simulink model "task_5_sim"  (R2022b)
settings: Solver=VariableStepAuto  StartTime=0.0  StopTime=20.0  RelTol=1e-3
model workspace (MAT data in the model file):
  C0 = [1  0  0  0  0  0; 0  1  0  0  0  0; 0  0  1  0  0  0; 0  0  0  1  0  0; 0  0  0  0  1  0; 0  0  0  0  0  1]
  D0 = [0  0; 0  0; 0  0; 0  0; 0  0; 0  0]
values from neighbouring files (symbols this model uses):
  KTld5_1 = real(getLQRController(ATld, BTld, Q, R))    [task5.m]
  L5_1 = K5_1'    [task5.m]
  r = -1/10*C*inv(A)*B*[-0.5+(a-b)/20; 0.1+(b-c)/(a+d+10)]    [task5.m]
undefined symbols (not defined in the file or in its folder): A, B, C
settings Model: Creator=小灰  LastModifiedBy=小灰

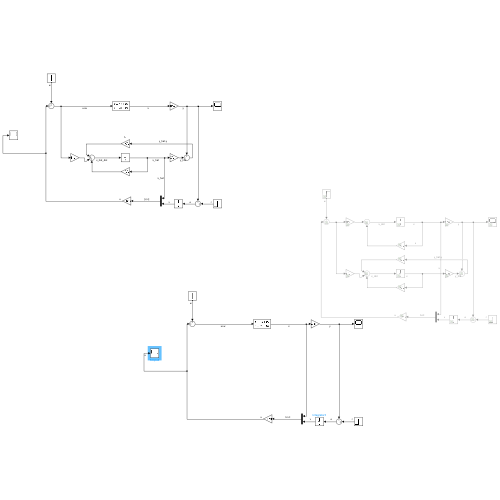
[thumbnail: Simulink's stored preview of the top-level diagram]
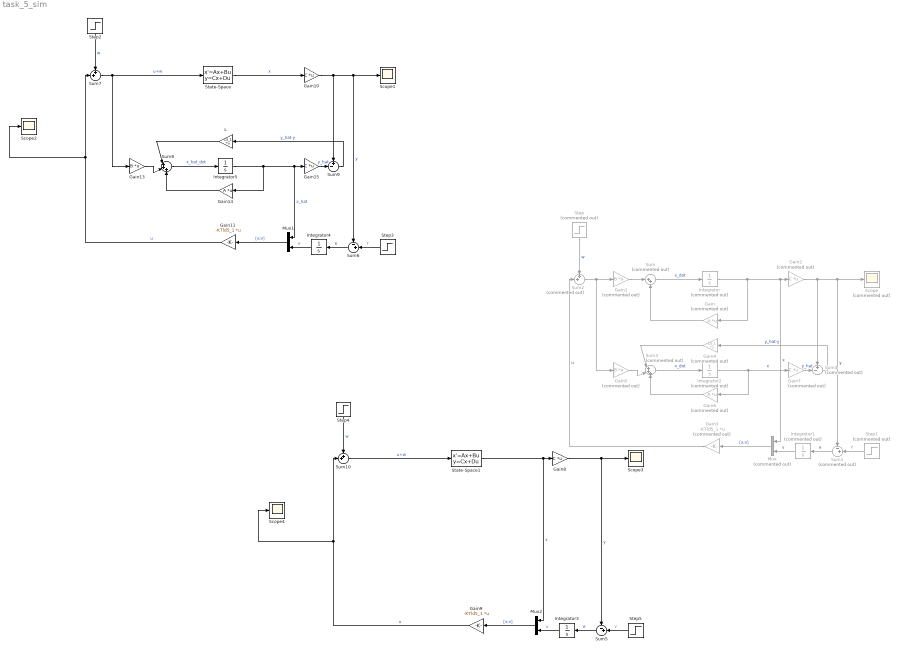
== system task_5_sim ==
  Gain : Gain  Commented=on  Gain=A  Multiplication=Matrix(K*u)
  Gain1 : Gain  Commented=on  Gain=B  Multiplication=Matrix(K*u)
  Gain10 : Gain  Gain=C  Multiplication=Matrix(K*u)
  Gain11 : Gain  Gain=-KTld5_1  Multiplication=Matrix(K*u)
  Gain13 : Gain  Gain=B  Multiplication=Matrix(K*u)
  Gain14 : Gain  Gain=A  Multiplication=Matrix(K*u)
  Gain15 : Gain  Gain=C  Multiplication=Matrix(K*u)
  Gain2 : Gain  Commented=on  Gain=C  Multiplication=Matrix(K*u)
  Gain3 : Gain  Commented=on  Gain=-KTld5_1  Multiplication=Matrix(K*u)
  Gain4 : Gain  Commented=on  Gain=L5_1  Multiplication=Matrix(K*u)
  Gain5 : Gain  Commented=on  Gain=B  Multiplication=Matrix(K*u)
  Gain6 : Gain  Commented=on  Gain=A  Multiplication=Matrix(K*u)
  Gain7 : Gain  Commented=on  Gain=C  Multiplication=Matrix(K*u)
  Gain8 : Gain  Gain=C  Multiplication=Matrix(K*u)
  Gain9 : Gain  Gain=-KTld5_1  Multiplication=Matrix(K*u)
  Integrator : Integrator  Commented=on
  Integrator1 : Integrator  Commented=on
  Integrator2 : Integrator  Commented=on
  Integrator3 : Integrator
  Integrator4 : Integrator
  Integrator5 : Integrator
  L : Gain  Gain=L5_1  Multiplication=Matrix(K*u)
  Mux : Mux  Commented=on  Inputs=2
  Mux1 : Mux  Inputs=2
  Mux2 : Mux  Inputs=2
  Scope : Scope  Commented=on
  Scope{1..4} (4 alike) : Scope
  State-Space : StateSpace  A=A  B=B  C=C0  D=D0  InitialCondition=0
  State-Space1 : StateSpace  A=A  B=B  C=C0  D=D0  InitialCondition=0
  Step : Step  Commented=on  Time=10  Before=[0;0]  After=[0;0]  SampleTime=0
  Step1 : Step  Commented=on  After=[0;1;0]  SampleTime=0
  Step2 : Step  Time=10  Before=[0;0]  After=0  SampleTime=0
  Step3 : Step  After=r  SampleTime=0
  Step4 : Step  Time=10  Before=[0;0]  After=0  SampleTime=0
  Step5 : Step  After=r  SampleTime=0
  Sum : Sum  Commented=on  Inputs=|++
  Sum1 : Sum  Commented=on  Inputs=-+|
  Sum10 : Sum  Inputs=++|
  Sum2 : Sum  Commented=on  Inputs=++|
  Sum3 : Sum  Commented=on  Inputs=|+++
  Sum4 : Sum  Commented=on  Inputs=+-|
  Sum5 : Sum  Inputs=-+|
  Sum6 : Sum  Inputs=-+|
  Sum7 : Sum  Inputs=++|
  Sum8 : Sum  Inputs=|+++
  Sum9 : Sum  Inputs=+-|
  wires:
  Sum/1 -> Integrator/1  "x_dot"
  Integrator/1 -> Gain/1, Mux/1, Gain2/1  "x"
  Gain2/1 -> Sum1/1, Scope/1, Sum4/1  "y"
  Mux/1 -> Gain3/1  "[x;v]"
  Sum1/1 -> Integrator1/1  "e"
  Integrator1/1 -> Mux/2  "v"
  Step/1 -> Sum2/1  "w"
  Gain3/1 -> Sum2/2  "u"
  Gain1/1 -> Sum/1
  Sum2/1 -> Gain5/1, Gain1/1
  Gain/1 -> Sum/2
  Step1/1 -> Sum1/2  "r"
  Sum3/1 -> Integrator2/1  "x_dot"
  Integrator2/1 -> Gain6/1, Gain7/1  "x"
  Gain7/1 -> Sum4/2  "y_hat"
  Sum4/1 -> Gain4/1  "y_hat-y"
  Gain6/1 -> Sum3/3
  Gain5/1 -> Sum3/2
  Gain4/1 -> Sum3/1
  L/1 -> Sum8/1
  Gain15/1 -> Sum9/2  "y_hat"
  Gain14/1 -> Sum8/3
  Sum9/1 -> L/1  "y_hat-y"
  Gain11/1 -> Scope2/1, Sum7/2  "u"
  Gain10/1 -> Sum6/1, Scope1/1, Sum9/1  "y"
  Sum7/1 -> State-Space/1, Gain13/1  "u+w"
  Step3/1 -> Sum6/2  "r"
  Integrator4/1 -> Mux1/2  "v"
  Mux1/1 -> Gain11/1  "[x;v]"
  Step2/1 -> Sum7/1  "w"
  Gain13/1 -> Sum8/2
  Integrator5/1 -> Gain14/1, Mux1/1, Gain15/1  "x_hat"
  Sum6/1 -> Integrator4/1  "e"
  Sum8/1 -> Integrator5/1  "x_hat_dot"
  State-Space/1 -> Gain10/1  "x"
  Sum5/1 -> Integrator3/1  "e"
  Integrator3/1 -> Mux2/2  "v"
  State-Space1/1 -> Mux2/1, Gain8/1  "x"
  Step5/1 -> Sum5/2  "r"
  Mux2/1 -> Gain9/1  "[x;v]"
  Step4/1 -> Sum10/1  "w"
  Sum10/1 -> State-Space1/1  "u+w"
  Gain8/1 -> Sum5/1, Scope3/1  "y"
  Gain9/1 -> Scope4/1, Sum10/2  "u"
